simulink model "test"  (R2013b)
settings: Solver=ode45  StartTime=0.0  StopTime=10.0  RelTol=1e-3
libraries: xbsIndex_r4 x20, xps_library x1
settings Model: Creator=root  LastModifiedBy=root

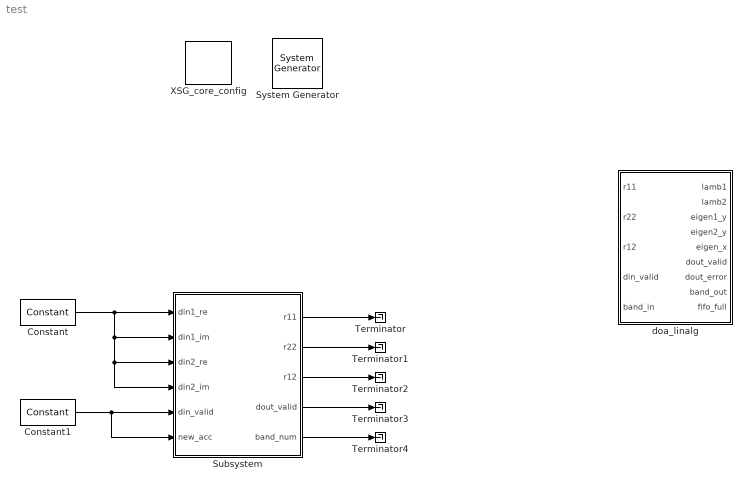
== system test ==
  " System Generator" : xbsIndex_r4/ System Generator  Tag=genX  xilinxfamily=Kintex7  part=xc7k325t  speed=-3  package=fbg676  synthesis_tool=XST  clock_wrapper=Clock Enables  directory=./netlist  proj_type=Project Navigator  Synth_file=XST Defaults  Impl_file=ISE Defaults  testbench=off  simulink_period=1  sysclk_period=10  dcm_input_clock_period=10  incr_netlist=off  trim_vbits=Everywhere in SubSystem  dbl_ovrd=According to Block Masks  core_generation=According to Block Masks  run_coregen=off  deprecated_control=off  eval_field=0  block_type=sysgen
  Constant : xbsIndex_r4/Constant  const=1  gui_display_data_type=Fixed-point  arith_type=Unsigned  n_bits=18*4  bin_pt=0  preci_type=Single  exp_width=8  frac_width=24  explicit_period=on  period=1  equ=P=C  opselect=C  inp2=PCIN>>17  opr=+  inp1=P  carry=CIN  dbl_ovrd=off  block_type=constant
  Constant1 : xbsIndex_r4/Constant  const=1  gui_display_data_type=Boolean  arith_type=Boolean  n_bits=18*4  bin_pt=0  preci_type=Single  exp_width=8  frac_width=24  explicit_period=on  period=1  equ=P=C  opselect=C  inp2=PCIN>>17  opr=+  inp1=P  carry=CIN  dbl_ovrd=off  block_type=constant
  Subsystem : Subsystem  mask{din_width=18, din_point=17, parallel=4, vector_len=2048, bands=8, pre_acc_delay=2, pre_acc_shift=0, acc_width=20, acc_point=10, dout_width=32}
      mask prompts: din_width "din width"; din_point "din point"; vector_len "vector lenght"; pre_acc_delay "pre acc delay"; pre_acc_shift "pre acc shift"; acc_width "accumulation input width"; acc_point "accumulation input point"; dout_width "output width"
  Terminator{,1..4} (5 alike) : Terminator
  XSG_core_config : xps_library/XSG_core_config  Tag=xps:xsg  hw_sys=ROACH2:sx475t  clk_src=sys_clk  ROACH_clk_src=sys_clk  ROACH2_clk_src=sys_clk  MKDIG_clk_src=sys_clk  clk_rate=100  sample_period=1  synthesis_tool=XST
  doa_linalg : Subsystem  mask{din_width=32, din_point=10, sqrt_width=8, dout_width=15, dout_point=0, bands=8, fifo_depth=8}
      mask prompts: din_width "din width"; din_point "din point"; sqrt_width "sqrt width"; dout_width "dout width"; dout_point "dout point"; fifo_depth "fifo depth"
  wires:
  Constant/1 -> Subsystem/3(din2_re), Subsystem/4(din2_im), Subsystem/2(din1_im), Subsystem/1(din1_re)
  Constant1/1 -> Subsystem/6(new_acc), Subsystem/5(din_valid)
  Subsystem/1(r11) -> Terminator/1
  Subsystem/2(r22) -> Terminator1/1
  Subsystem/3(r12) -> Terminator2/1
  Subsystem/4(dout_valid) -> Terminator3/1
  Subsystem/5(band_num) -> Terminator4/1

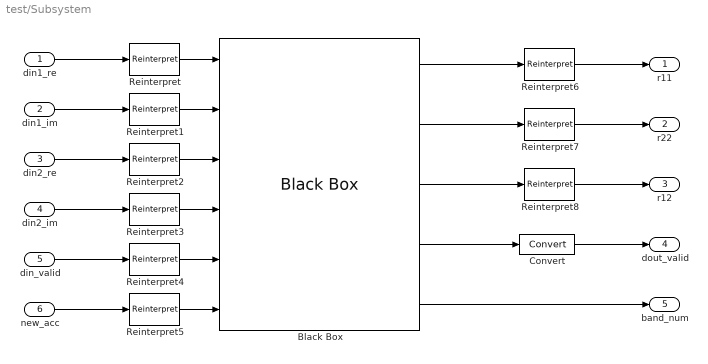
== system test/Subsystem ==
  din1_re : Inport
  din1_im : Inport  Port=2
  din2_re : Inport  Port=3
  din2_im : Inport  Port=4
  din_valid : Inport  Port=5
  new_acc : Inport  Port=6
  Black Box : xbsIndex_r4/Black Box  init_code=band_doa_no_la_config  sim_method=Inactive  verbose=off  block_type=blackbox2
  Convert : xbsIndex_r4/Convert  gui_display_data_type=Boolean  arith_type=Boolean  n_bits=3  bin_pt=0  float_type=Single  exp_bits=8  fraction_bits=24  quantization=Truncate  overflow=Wrap  en=off  latency=0  dbl_ovrd=off  pipeline=off  block_type=convert
      settings: block_version=11.4
  Reinterpret : xbsIndex_r4/Reinterpret  force_arith_type=on  arith_type=Unsigned  force_bin_pt=on  bin_pt=acc_point  block_type=reinterpret
  Reinterpret{1..5} (5 alike) : xbsIndex_r4/Reinterpret  force_arith_type=on  arith_type=Unsigned  force_bin_pt=on  bin_pt=0  block_type=reinterpret
  Reinterpret6 : xbsIndex_r4/Reinterpret  force_arith_type=on  arith_type="Signed  (2's comp)"  force_bin_pt=on  bin_pt=0  block_type=reinterpret
  Reinterpret7 : xbsIndex_r4/Reinterpret  force_arith_type=on  arith_type="Signed  (2's comp)"  force_bin_pt=on  bin_pt=acc_point  block_type=reinterpret
  Reinterpret8 : xbsIndex_r4/Reinterpret  force_arith_type=on  arith_type="Signed  (2's comp)"  force_bin_pt=on  bin_pt=acc_point  block_type=reinterpret
  r11 : Outport
  r22 : Outport  Port=2
  r12 : Outport  Port=3
  dout_valid : Outport  Port=4
  band_num : Outport  Port=5
  wires:
  din1_re/1 -> Reinterpret/1
  din1_im/1 -> Reinterpret1/1
  din_valid/1 -> Reinterpret4/1
  din2_im/1 -> Reinterpret3/1
  din2_re/1 -> Reinterpret2/1
  Black Box/1 -> Reinterpret6/1
  new_acc/1 -> Reinterpret5/1
  Black Box/3 -> Reinterpret8/1
  Black Box/5 -> band_num/1
  Black Box/4 -> Convert/1
  Black Box/2 -> Reinterpret7/1
  Reinterpret/1 -> Black Box/1
  Reinterpret1/1 -> Black Box/2
  Reinterpret3/1 -> Black Box/4
  Reinterpret2/1 -> Black Box/3
  Reinterpret5/1 -> Black Box/6
  Reinterpret4/1 -> Black Box/5
  Reinterpret6/1 -> r11/1
  Reinterpret7/1 -> r22/1
  Reinterpret8/1 -> r12/1
  Convert/1 -> dout_valid/1

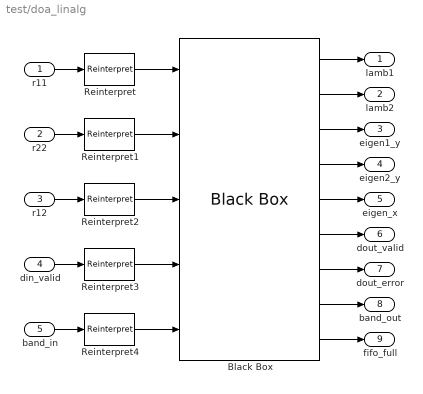
== system test/doa_linalg ==
  r11 : Inport
  r22 : Inport  Port=2
  r12 : Inport  Port=3
  din_valid : Inport  Port=4
  band_in : Inport  Port=5
  Black Box : xbsIndex_r4/Black Box  init_code=quad_eigen_iterative_config  sim_method=Inactive  verbose=off  block_type=blackbox2
  Reinterpret{,1..4} (5 alike) : xbsIndex_r4/Reinterpret  force_arith_type=on  arith_type=Unsigned  force_bin_pt=on  bin_pt=0  block_type=reinterpret
  lamb1 : Outport
  lamb2 : Outport  Port=2
  eigen1_y : Outport  Port=3
  eigen2_y : Outport  Port=4
  eigen_x : Outport  Port=5
  dout_valid : Outport  Port=6
  dout_error : Outport  Port=7
  band_out : Outport  Port=8
  fifo_full : Outport  Port=9
  wires:
  Black Box/8 -> band_out/1
  Black Box/9 -> fifo_full/1
  band_in/1 -> Reinterpret4/1
  r12/1 -> Reinterpret2/1
  din_valid/1 -> Reinterpret3/1
  Black Box/2 -> lamb2/1
  Black Box/7 -> dout_error/1
  r22/1 -> Reinterpret1/1
  Black Box/3 -> eigen1_y/1
  Black Box/4 -> eigen2_y/1
  Black Box/6 -> dout_valid/1
  r11/1 -> Reinterpret/1
  Black Box/1 -> lamb1/1
  Black Box/5 -> eigen_x/1
  Reinterpret/1 -> Black Box/1
  Reinterpret1/1 -> Black Box/2
  Reinterpret2/1 -> Black Box/3
  Reinterpret3/1 -> Black Box/4
  Reinterpret4/1 -> Black Box/5
